simulink model "rtwdemo_async"  (Simulink 6.0)
settings: Solver=FixedStepDiscrete  SolverMode=MultiTasking  StartTime=0.0  StopTime=0.5  RelTol=1e-3  AbsTol=1e-6  SampleTimeConstraint=Specified
PreLoadFcn:
  | width = 160;
undefined symbols (not defined in the file or in its folder): DiscIntNeverNeededParam
libraries: vxlib1 x2, rtwdemowidgets x2, simulink x1
settings Model: Creator=The MathWorks Inc.  LastModifiedBy=batserve  ExtModeTrigMode=oneshot  ExtModeArmWhenConnect=off  ExtModeAutoUpdateStatusClock=off
settings SolverCC: AutoInsertRateTranBlk=on
settings MATStruct: SampleTime=1/60  Offset=0  Priority=[41.0]
settings DataIOCC: LimitDataPoints=off  SaveOutput=off  SaveTime=off  SignalLoggingName=sigsOut
settings OptimizationCC: InlineParams=on  EnforceIntegerDowncast=off  StateBitsets=on  DataBitsets=on  UseTempVars=on
settings DebuggingCC: CheckExecutionContextPreStartOutputMsg=on  CheckExecutionContextRuntimeOutputMsg=on  SolverPrmCheckMsg=none  InheritedTsInSrcMsg=none  IntegerOverflowMsg=none  UnconnectedInputMsg=none  UnconnectedOutputMsg=none  UnconnectedLineMsg=none
settings ModelReferenceCC: UpdateModelReferenceTargets=IfOutOfDate
settings RTWCC: TLCOptions=-p0 -aWarnNonSaturatedBlocks=0  GenCodeOnly=on  GenerateReport=on  RTWVerbose=off  ProcessScript=grt_make_rtw_hook  LaunchReport=on
settings CodeAppCC: ForceParamTrailComments=on  PrefixModelToSubsysFcnNames=off
settings GRTTargetCC: MatFileLogging=off

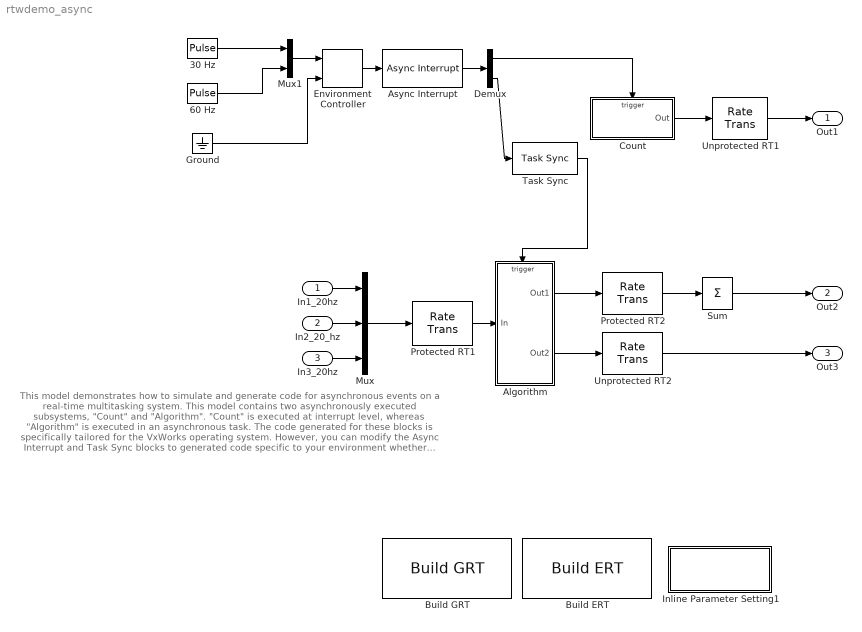
== system rtwdemo_async ==
  note: This model demonstrates how to simulate and generate code for asynchronous events on a real-time multitasking
      | system.  This model contains two asynchronously executed subsystems, "Count" and "Algorithm". "Count"
      | is executed at interrupt level, whereas "Algorithm" is executed in an asynchronous task. The code generated
      | for these blocks is specifically tailored for the VxWorks operating system.  However, you can modify the
      | Async Interrupt and Task Sync blocks to generated code specific to your environment whether you're using
      | an operating system or not.
  In1_20hz : Inport  Port=1  PortDimensions=20  SampleTime=1/20  LatchInput=off
  In2_20_hz : Inport  Port=2  PortDimensions=20  SampleTime=1/20  LatchInput=off
  In3_20hz : Inport  Port=3  PortDimensions=20  SampleTime=1/20  LatchInput=off
  30 Hz : DiscretePulseGenerator  SampleTime=1/30  VectorParams1D=off
  60 Hz : DiscretePulseGenerator  Period=4  PulseWidth=2  SampleTime=1/60
  Algorithm : Subsystem  TreatAsAtomicUnit=on  PropExecContextAcrossSSBoundary=on  RTWFcnName=Algorithm  RTWFileName=Algorithm
      settings: RTWFcnNameOpts=User specified  RTWFileNameOpts=User specified
  Async Interrupt : vxlib1/Async Interrupt  irqnumbers=[1 2]  irqoffsets=[192 193]  irqpriorities=[10 11]  irqpreempts=[0 1]  tickres=1/60  showinput=on
  Build ERT : rtwdemowidgets/Build ERT  attrib_overrides={}
  Build GRT : rtwdemowidgets/Build GRT  attrib_overrides={}
  Count : Subsystem  TreatAsAtomicUnit=on  PropExecContextAcrossSSBoundary=on  RTWFcnName=Count  RTWFileName=Count
      settings: RTWFcnNameOpts=User specified  RTWFileNameOpts=User specified
  Demux : Demux  Outputs=2
  Environment Controller : simulink/Signal Routing/Environment Controller
  Ground : Ground
  Inline Parameter Setting1 : Subsystem  Orientation=up  PropExecContextAcrossSSBoundary=on
      settings: OpenFcn=m=get_param(bdroot,'name'); eval([m,'([],[],[],''compile'');']); eval([m,'([],[],[],''term'');']);
      mask Display: disp(sprintf('Display Sample\nTime Colors\n(double-click)'))
  Mux : Mux  Inputs=3
  Mux1 : Mux  Inputs=2
  Protected RT1 : RateTransition  Deterministic=off  OutPortSampleTime=1/20
  Protected RT2 : RateTransition  Deterministic=off  OutPortSampleTime=1/20
  Sum : Sum  Inputs=1  SaturateOnIntegerOverflow=on  InputSameDT=on
  Task Sync : vxlib1/Task Sync  taskname=Task0  taskpriority=50  taskstacksize=8192  parentmanaget=on  tickres=1/60
  Unprotected RT1 : RateTransition  Integrity=off  OutPortSampleTime=1/20
  Unprotected RT2 : RateTransition  Integrity=off  OutPortSampleTime=1/20
  Out1 : Outport
  Out2 : Outport  Port=2
  Out3 : Outport  Port=3
  wires:
  Protected RT1/1 -> Algorithm/1(In)
  Mux/1 -> Protected RT1/1
  Algorithm/1(Out1) -> Protected RT2/1
  Protected RT2/1 -> Sum/1
  Sum/1 -> Out2/1
  Task Sync/1 -> Algorithm/Trigger
  Algorithm/2(Out2) -> Unprotected RT2/1
  Unprotected RT2/1 -> Out3/1
  Count/1(Out) -> Unprotected RT1/1
  Unprotected RT1/1 -> Out1/1
  In1_20hz/1 -> Mux/1
  In2_20_hz/1 -> Mux/2
  In3_20hz/1 -> Mux/3
  60 Hz/1 -> Mux1/2
  Environment Controller/1 -> Async Interrupt/1
  Ground/1 -> Environment Controller/2
  30 Hz/1 -> Mux1/1
  Mux1/1 -> Environment Controller/1
  Async Interrupt/1 -> Demux/1
  Demux/1 -> Count/Trigger
  Demux/2 -> Task Sync/1

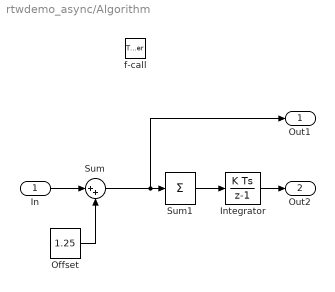
== system rtwdemo_async/Algorithm ==
  In : Inport  Port=1  LatchInput=off
  f-call : TriggerPort  TriggerType=function-call
  Integrator : DiscreteIntegrator  SampleTime=-1  SaturateOnIntegerOverflow=on  ICPrevOutput=DiscIntNeverNeededParam  ICPrevScaledInput=DiscIntNeverNeededParam
  Offset : Constant  Value=1.25
  Sum : Sum  Inputs=|++
  Sum1 : Sum  Inputs=1  SaturateOnIntegerOverflow=on  InputSameDT=on
  Out1 : Outport  InitialOutput=0
  Out2 : Outport  Port=2  InitialOutput=0
  wires:
  In/1 -> Sum/1
  Sum/1 -> Sum1/1, Out1/1
  Sum1/1 -> Integrator/1
  Integrator/1 -> Out2/1
  Offset/1 -> Sum/2

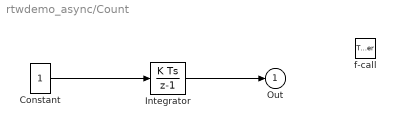
== system rtwdemo_async/Count ==
  f-call : TriggerPort  TriggerType=function-call
  Constant : Constant
  Integrator : DiscreteIntegrator  SampleTime=-1  SaturateOnIntegerOverflow=on  ICPrevOutput=DiscIntNeverNeededParam  ICPrevScaledInput=DiscIntNeverNeededParam
  Out : Outport  InitialOutput=0
  wires:
  Constant/1 -> Integrator/1
  Integrator/1 -> Out/1

== system rtwdemo_async/Inline Parameter Setting1 ==
